simulink model "HANcoder_E407_CAN_COMM_TEST"  (R2018b)
settings: Solver=FixedStepDiscrete  StartTime=0.0  StopTime=1  FixedStep=0.01  RelTol=1e-3
PreLoadFcn:
  | librarySetup
  | eval([bdroot,'_startup']) %Calling [modelName]_startup.m
values from neighbouring files (symbols this model uses):
  HANtuneOverride = Simulink.Parameter    [HANcoder_E407_CAN_COMM_TEST_startup.m]    (also in HANcoder_E407_TTA_Controller_v3_startup.m; HANcoder_E407_TTA_Template_startup.m; HANcoder_Olimexino_startup.m)
  ID_CAN1_const = 24    [HANcoder_E407_CAN_COMM_TEST_startup.m]
  ID_CAN2_const = 24    [HANcoder_E407_CAN_COMM_TEST_startup.m]
  precision_CAN1 = Simulink.Parameter    [HANcoder_E407_CAN_COMM_TEST_startup.m]
  precision_CAN2 = Simulink.Parameter    [HANcoder_E407_CAN_COMM_TEST_startup.m]
  Rx_ID_CAN1 = Simulink.Parameter    [HANcoder_E407_CAN_COMM_TEST_startup.m]
  Rx_ID_CAN2 = Simulink.Parameter    [HANcoder_E407_CAN_COMM_TEST_startup.m]
  Tx_Buffer_1_CAN1 = Simulink.Parameter    [HANcoder_E407_CAN_COMM_TEST_startup.m]
  Tx_Buffer_1_CAN2 = Simulink.Parameter    [HANcoder_E407_CAN_COMM_TEST_startup.m]
  Tx_Buffer_2_CAN1 = Simulink.Parameter    [HANcoder_E407_CAN_COMM_TEST_startup.m]
  Tx_Buffer_2_CAN2 = Simulink.Parameter    [HANcoder_E407_CAN_COMM_TEST_startup.m]
  Tx_Buffer_3_CAN1 = Simulink.Parameter    [HANcoder_E407_CAN_COMM_TEST_startup.m]
  Tx_Buffer_3_CAN2 = Simulink.Parameter    [HANcoder_E407_CAN_COMM_TEST_startup.m]
  Tx_Buffer_4_CAN1 = Simulink.Parameter    [HANcoder_E407_CAN_COMM_TEST_startup.m]
  Tx_Buffer_4_CAN2 = Simulink.Parameter    [HANcoder_E407_CAN_COMM_TEST_startup.m]
  Tx_Buffer_5_CAN1 = Simulink.Parameter    [HANcoder_E407_CAN_COMM_TEST_startup.m]
  Tx_Buffer_5_CAN2 = Simulink.Parameter    [HANcoder_E407_CAN_COMM_TEST_startup.m]
  Tx_Buffer_6_CAN1 = Simulink.Parameter    [HANcoder_E407_CAN_COMM_TEST_startup.m]
  Tx_Buffer_6_CAN2 = Simulink.Parameter    [HANcoder_E407_CAN_COMM_TEST_startup.m]
  Tx_Buffer_7_CAN1 = Simulink.Parameter    [HANcoder_E407_CAN_COMM_TEST_startup.m]
  Tx_Buffer_7_CAN2 = Simulink.Parameter    [HANcoder_E407_CAN_COMM_TEST_startup.m]
  Tx_Buffer_8_CAN1 = Simulink.Parameter    [HANcoder_E407_CAN_COMM_TEST_startup.m]
  Tx_Buffer_8_CAN2 = Simulink.Parameter    [HANcoder_E407_CAN_COMM_TEST_startup.m]
  Tx_ID_CAN1 = Simulink.Parameter    [HANcoder_E407_CAN_COMM_TEST_startup.m]
  Tx_ID_CAN2 = Simulink.Parameter    [HANcoder_E407_CAN_COMM_TEST_startup.m]
  Tx_Max_CAN1 = Simulink.Parameter    [HANcoder_E407_CAN_COMM_TEST_startup.m]
  Tx_Max_CAN2 = Simulink.Parameter    [HANcoder_E407_CAN_COMM_TEST_startup.m]
  Tx_Min_CAN1 = Simulink.Parameter    [HANcoder_E407_CAN_COMM_TEST_startup.m]
  Tx_Min_CAN2 = Simulink.Parameter    [HANcoder_E407_CAN_COMM_TEST_startup.m]
libraries: hdlsllib x48, HANcoder_STM32_Target x13, simulink x2
(part 1 of 3)
CloseFcn:
  | rtwprivate ssgencode ModelCloseRequest mytest
settings Model: Creator=Jason van Kolfschoten  LastModifiedBy=Diego
settings SolverCC: PositivePriorityOrder=on
settings DataIOCC: LimitDataPoints=on  SaveFormat=Array  SignalLoggingSaveFormat=ModelDataLogs  SaveOutput=off  SaveTime=off
settings OptimizationCC: BlockReduction=off  DefaultParameterBehavior=Inlined  InlineInvariantSignals=on  ExpressionDepthLimit=2147483647  StateBitsets=on  DataBitsets=on  ZeroExternalMemoryAtStartup=off  ZeroInternalMemoryAtStartup=off  InitFltsAndDblsToZero=on  NoFixptDivByZeroProtection=on  EfficientFloat2IntCast=on  LifeSpan=inf
settings DebuggingCC: SaveWithDisabledLinksMsg=none  SaveWithParameterizedLinksMsg=none  CheckSSInitialOutputMsg=off  UnderspecifiedInitializationDetection=Classic  MergeDetectMultiDrivingBlocksExec=none  SignalResolutionControl=TryResolveAll  SolverPrmCheckMsg=warning  InheritedTsInSrcMsg=none  MultiTaskDSMMsg=warning  MultiTaskCondExecSysMsg=none  ParameterPrecisionLossMsg=none  FcnCallInpInsideContextMsg=warning  StateNameClashWarn=warning  SFUnexpectedBacktrackingDiag=warning  SFNoUnconditionalDefaultTransitionDiag=warning  SFExecutionAtInitializationDiag=none
settings HardwareCC: ProdBitPerPointer=32  ProdBitPerSizeT=32  ProdBitPerPtrDiffT=32  ProdLargestAtomicFloat=None  ProdIntDivRoundTo=Undefined  ProdWordSize=32  ProdHWDeviceType=Generic->32-bit Embedded Processor  TargetEndianess=LittleEndian  TargetHWDeviceType=Infineon->TriCore
settings ModelReferenceCC: PropagateSignalLabelsOutOfModel=off
settings SFSimCC: SimUseLocalCustomCode=off  MATLABDynamicMemAlloc=off
settings RTWCC: SystemTargetFile=ert.tlc  MakeCommand=make_rtw SHELL= HANcoder_PORTABLE=1 HANcoder_BOOTLOADER=1  TemplateMakefile=STM32_E407_gcc.tmf  Description=Real-Time Workshop Embedded Coder (no auto configuration)  RTWUseLocalCustomCode=off
settings CodeAppCC: ForceParamTrailComments=on  IgnoreCustomStorageClasses=off  SimulinkDataObjDesc=on  CustomSymbolStrGlobalVar=rt$N$M  CustomSymbolStrType=$N$M  CustomSymbolStrFcn=$N$M$F  CustomSymbolStrMacro=$N$M  InsertBlockDesc=on  StateflowObjectComments=on  InternalIdentifier=Classic
settings ERTTargetCC: TargetFcnLib=ansi_tfl_tmw.mat  MultiwordLength=2048  IncludeMdlTerminateFcn=off  SuppressErrorStatus=on  SupportNonFinite=off  GenerateASAP2=on  InlinedParameterPlacement=NonHierarchical  ERTCustomFileTemplate=example_file_process.tlc  ConvertIfToSwitch=off  SuppressUnreachableDefaultCases=off
settings ConfigComp: CovMetricSettings=dw  CovHtmlReporting=on  CovSaveCumulativeToWorkspaceVar=on  CovSaveSingleToWorkspaceVar=on  CovExternalEMLEnable=off  DVMaxProcessTime=600  DVDisplayUnsatisfiableObjectives=on  DVAutomaticStubbing=off  DVModelCoverageObjectives=MCDC  DVMaxTestCaseSteps=500  DVTestSuiteOptimization=CombinedObjectives  DVDetectActiveLogic=on  DVSaveHarnessModel=on

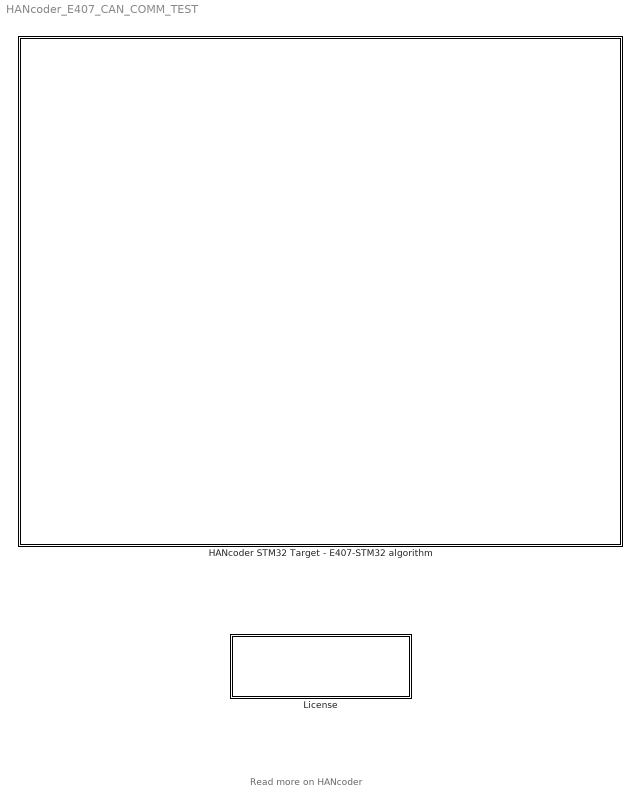
== system HANcoder_E407_CAN_COMM_TEST ==
  note: Read more on HANcoder
  HANcoder STM32 Target - E407-STM32 algorithm : Subsystem  mask(TopLevelSubsystem){}
      settings: CopyFcn=HANcoderChecks('Copy');  NameChangeFcn=HANcoderChecks('NameChangeE407');  MoveFcn=HANcoderChecks('MoveE407');
      mask Display: image(imread('STM32_E407_HAN.jpg'))
  License : Subsystem  mask(License){}
      settings: NameChangeFcn=HANcoderChecks('NameChangeLicenseBlock');  OpenFcn=winopen('License.pdf')  MoveFcn=HANcoderChecks('MoveLicenseBlock');
      mask Display: disp(['End-User License Agreement\n','please read before use']);

== system HANcoder_E407_CAN_COMM_TEST/HANcoder STM32 Target - E407-STM32 algorithm ==
  note: Board with ID 2 receives the messages
  note: Board with ID1 sends a message when the WKUP Button is pressed
  note: Basic principle:
      |
      | - Board id 1 sends a count over both CAN buses.
      |
      | - Other board receives the messages.
  note: Template model
  AND1 : Logic  IconShape=distinctive  AllPortsSameDT=off  OutDataTypeStr=boolean
  AND3 : Logic  IconShape=distinctive  AllPortsSameDT=off  OutDataTypeStr=boolean
  Algorithm : Subsystem
  Base Sample Time config : HANcoder_STM32_Target/STM32-E407/System Config/Base Sample Time config  Tag=HANcoder_TARGET_STM32_E407  Description=HANcoder Target STM32-E407 blockset version 1.0  baseSampleTime=10  extraStack=0
      settings: SourceProductName=HANcoder STM32 Target
  Build settings : HANcoder_STM32_Target/STM32-E407/System Config/Build settings  Tag=HANcoder_TARGET_STM32_E407  AutoASAP2add=on  AutoFlash=USB
      settings: SourceProductName=HANcoder STM32 Target
  CAN config : HANcoder_STM32_Target/STM32-E407/System Config/CAN config  Tag=HANcoder_TARGET_STM32_E407  txBufSize=64  evBufSize=8  canBus1=on  baudRate1=125  rxMask1=hex2dec('00000000')  rxCode1=hex2dec('00000000')  rxMode1=Receive only 11-bit message identifiers  canBus2=on  baudRate2=125  rxMask2=hex2dec('00000000')  rxCode2=hex2dec('00000000')  rxMode2=Receive only 11-bit message identifiers
      settings: SourceProductName=HANcoder STM32 Target
  Custom ID config : HANcoder_STM32_Target/STM32-E407/System Config/Custom ID config  Tag=HANcoder_TARGET_STM32_E407  softID=softwareID  softNUM=1
      settings: SourceProductName=HANcoder STM32 Target
  Data Store Memory : DataStoreMemory  DataStoreName=HANtuneOverride1  ReadBeforeWriteMsg=warning  WriteAfterWriteMsg=warning  WriteAfterReadMsg=warning  ShowAdditionalParam=off
  Digital Input : HANcoder_STM32_Target/STM32-E407/Digital Inputs/Digital Input  Tag=HANcoder_TARGET_STM32_E407  pinID=CON3 - D2 - 5V Tolerant  config=Pulldown  tsamp=-1
      settings: SourceProductName=HANcoder STM32 Target
  Digital Input1 : HANcoder_STM32_Target/STM32-E407/Digital Inputs/Digital Input  Tag=HANcoder_TARGET_STM32_E407  pinID=CON3 - D3 - 5V Tolerant  config=Pulldown  tsamp=-1
      settings: SourceProductName=HANcoder STM32 Target
  Inputs : Subsystem
  Outputs : Subsystem
  Rx CAN : Subsystem
  System information : Subsystem
  Tx CAN : Subsystem  TreatAsAtomicUnit=on
  XCP on CAN config : HANcoder_STM32_Target/STM32-E407/System Config/XCP on CAN config  Tag=HANcoder_TARGET_STM32_E407  Commented=on  canBus=CAN 1  croID=hex2dec('665')  dtoID=hex2dec('666')
      settings: SourceProductName=HANcoder STM32 Target
  XCP on USB config : HANcoder_STM32_Target/STM32-E407/System Config/XCP on USB config  Tag=HANcoder_TARGET_STM32_E407
      settings: SourceProductName=HANcoder STM32 Target
  wires:
  Inputs/1(Button) -> Algorithm/1(Button), AND1/1, AND3/1  "WKUP_button"
  Algorithm/1(LED) -> Outputs/1(LED)
  Digital Input/1 -> AND3/2  "sender_id"
  AND3/1 -> Tx CAN/Enable
  Digital Input1/1 -> AND1/2  "receiver_id"
  AND1/1 -> Rx CAN/Enable

== system HANcoder_E407_CAN_COMM_TEST/License ==

== system HANcoder_E407_CAN_COMM_TEST/HANcoder STM32 Target - E407-STM32 algorithm/Algorithm ==
  note: The button or the HANtuneOverride parameter
      | switches between the two frequencies.
  note: Here the algorithm can be placed. No hardware dependent blocks should be used here.
  note: Switch LED frequency when button is pressed
  Button : Inport
  10Hz Counter Limiter : simulink/Sources/Counter Limited  uplimit=1  tsamp=0.1
  5Hz Counter Limited : simulink/Sources/Counter Limited  uplimit=1  tsamp=0.2
  Constant : Constant  Value=HANtuneOverride  OutDataTypeStr=boolean
  Data Type Conversion : DataTypeConversion  OutDataTypeStr=boolean
  Logical Operator : Logic  Operator=OR  AllPortsSameDT=off  OutDataTypeStr=boolean
  Switch : Switch  Criteria=u2 > Threshold
  LED : Outport
  wires:
  Data Type Conversion/1 -> LED/1  "LedValue"
  5Hz Counter Limited/1 -> Switch/3
  Switch/1 -> Data Type Conversion/1
  Button/1 -> Logical Operator/2
  Logical Operator/1 -> Switch/2
  Constant/1 -> Logical Operator/1
  10Hz Counter Limiter/1 -> Switch/1

== system HANcoder_E407_CAN_COMM_TEST/HANcoder STM32 Target - E407-STM32 algorithm/Inputs ==
  note: The inputs and outputs are kept in a separate subsystem, this way the algorithm can easily be transferred to different hardware
  Digital Input : HANcoder_STM32_Target/STM32-E407/Digital Inputs/Digital Input  Tag=HANcoder_TARGET_STM32_E407  pinID=WKUP button  config=Pulldown  tsamp=-1
      settings: SourceProductName=HANcoder STM32 Target
  Button : Outport
  wires:
  Digital Input/1 -> Button/1

== system HANcoder_E407_CAN_COMM_TEST/HANcoder STM32 Target - E407-STM32 algorithm/Outputs ==
  note: The inputs and outputs are kept in a separate subsystem, this way the algorithm can easily be transferred to different hardware
  LED : Inport
  Digital Output : HANcoder_STM32_Target/STM32-E407/Digital Outputs/Digital Output  Tag=HANcoder_TARGET_STM32_E407  pinID=LED  config=Push pull  tsamp=-1
      settings: SourceProductName=HANcoder STM32 Target
  wires:
  LED/1 -> Digital Output/1

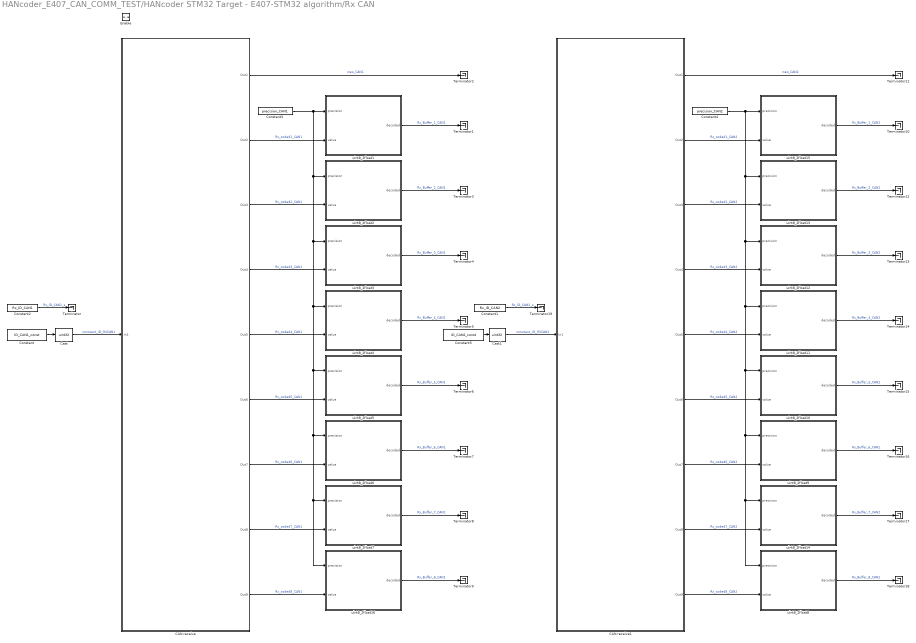
== system HANcoder_E407_CAN_COMM_TEST/HANcoder STM32 Target - E407-STM32 algorithm/Rx CAN ==
  Enable : EnablePort
  CAN receive : Subsystem  Tag=HANcoder_TARGET_STM32_E407  AncestorBlock=HANcoder_STM32_Target/STM32-E407/CAN/CAN/CAN receive  mask(CAN receive){canBus=CAN 1, outputNumber=8, dataType=uint8, byteOrder=off, tsamp=-1}
      mask prompts: canBus "CAN channel"; outputNumber "Output ports"; dataType "Output datatype"; byteOrder "Byte order: Checked = MSB first, unchecked = LSB first."; tsamp "Sample time"
      mask help:
      | Function
      | ==========
      | Receive the newest message from the specified CAN channel.
      |
      | Parameters
      | ==========
      | CAN channel:             The CAN channel to send the message on.
      | Output ports:             The amount of output ports
      | Output datatype:       The datatype of the output ports
      | Byte order:                 Select MSB or LSB first
      | Sample time:              -1 or divisible by base sample time [seconds]
      |
      | Input
      | ==========
      | Port 1:                       CAN ID(uint32) in hexadecimal ie: hex2dec('0a')
      |
      | Output
      | ==========
      | Port 1:                       Checks for new message(int8)
      | Port 2..9                     Message data
      mask init:
      | sfcn_can_receive_mcb(canBus, outputNumber, dataType, byteOrder)
      settings: MoveFcn=drawLogos
      mask Help: web('sfcn_can_receive.html');
      mask TypeOptions canBus: CAN 1 | CAN 2
      mask TypeOptions dataType: int8 | uint8 | int16 | uint16 | int32 | uint32 | boolean
      mask Display:
      | fprintf('Receive on\nCAN %x', canBus);
      | port_label('output', 1, 'new');
      | port_label('input', 1, 'ID');patch([335 341 341],[8 14 2],[1 0 0]);patch([343 343 349],[14 2 8],[0 0 0.35]);
  CAN receive1 : Subsystem  Tag=HANcoder_TARGET_STM32_E407  AncestorBlock=HANcoder_STM32_Target/STM32-E407/CAN/CAN/CAN receive  mask(CAN receive){canBus=CAN 2, outputNumber=8, dataType=uint8, byteOrder=off, tsamp=-1}
      mask prompts: canBus "CAN channel"; outputNumber "Output ports"; dataType "Output datatype"; byteOrder "Byte order: Checked = MSB first, unchecked = LSB first."; tsamp "Sample time"
      mask help:
      | Function
      | ==========
      | Receive the newest message from the specified CAN channel.
      |
      | Parameters
      | ==========
      | CAN channel:             The CAN channel to send the message on.
      | Output ports:             The amount of output ports
      | Output datatype:       The datatype of the output ports
      | Byte order:                 Select MSB or LSB first
      | Sample time:              -1 or divisible by base sample time [seconds]
      |
      | Input
      | ==========
      | Port 1:                       CAN ID(uint32) in hexadecimal ie: hex2dec('0a')
      |
      | Output
      | ==========
      | Port 1:                       Checks for new message(int8)
      | Port 2..9                     Message data
      mask init:
      | sfcn_can_receive_mcb(canBus, outputNumber, dataType, byteOrder)
      settings: MoveFcn=drawLogos
      mask Help: web('sfcn_can_receive.html');
      mask TypeOptions canBus: CAN 1 | CAN 2
      mask TypeOptions dataType: int8 | uint8 | int16 | uint16 | int32 | uint32 | boolean
      mask Display:
      | fprintf('Receive on\nCAN %x', canBus);
      | port_label('output', 1, 'new');
      | port_label('input', 1, 'ID');patch([335 341 341],[8 14 2],[1 0 0]);patch([343 343 349],[14 2 8],[0 0 0.35]);
  Cast : DataTypeConversion  OutDataTypeStr=uint32
  Cast1 : DataTypeConversion  OutDataTypeStr=uint32
  Constant : Constant  Value=ID_CAN1_const
  Constant1 : Constant  Value=Rx_ID_CAN2  OutDataTypeStr=uint32
  Constant2 : Constant  Value=Rx_ID_CAN1  OutDataTypeStr=uint32
  Constant3 : Constant  Value=precision_CAN1
  Constant4 : Constant  Value=precision_CAN2
  Constant5 : Constant  Value=ID_CAN2_const
  Terminator{,1..19} (20 alike) : Terminator
  uint8_2float1 : Subsystem
  uint8_2float10 : Subsystem
  uint8_2float11 : Subsystem
  uint8_2float12 : Subsystem
  uint8_2float13 : Subsystem
  uint8_2float14 : Subsystem
  uint8_2float15 : Subsystem
  uint8_2float16 : Subsystem
  uint8_2float2 : Subsystem
  uint8_2float3 : Subsystem
  uint8_2float4 : Subsystem
  uint8_2float5 : Subsystem
  uint8_2float6 : Subsystem
  uint8_2float7 : Subsystem
  uint8_2float8 : Subsystem
  uint8_2float9 : Subsystem
  wires:
  Constant/1 -> Cast/1
  CAN receive/1(Out1) -> Terminator2/1  "new_CAN1"
  Constant3/1 -> uint8_2float1/1(precision), uint8_2float2/1(precision), uint8_2float16/1(precision), uint8_2float7/1(precision), uint8_2float6/1(precision), uint8_2float5/1(precision), uint8_2float4/1(precision), uint8_2float3/1(precision)
  CAN receive/2(Out2) -> uint8_2float1/2(value)  "Rx_coded1_CAN1"
  CAN receive/3(Out3) -> uint8_2float2/2(value)  "Rx_coded2_CAN1"
  uint8_2float1/1(decoded) -> Terminator1/1  "Rx_Buffer_1_CAN1"
  uint8_2float2/1(decoded) -> Terminator3/1  "Rx_Buffer_2_CAN1"
  uint8_2float3/1(decoded) -> Terminator4/1  "Rx_Buffer_3_CAN1"
  uint8_2float4/1(decoded) -> Terminator5/1  "Rx_Buffer_4_CAN1"
  uint8_2float5/1(decoded) -> Terminator6/1  "Rx_Buffer_5_CAN1"
  uint8_2float6/1(decoded) -> Terminator7/1  "Rx_Buffer_6_CAN1"
  uint8_2float7/1(decoded) -> Terminator8/1  "Rx_Buffer_7_CAN1"
  uint8_2float16/1(decoded) -> Terminator9/1  "Rx_Buffer_8_CAN1"
  CAN receive/9(Out9) -> uint8_2float16/2(value)  "Rx_coded8_CAN1"
  CAN receive/8(Out8) -> uint8_2float7/2(value)  "Rx_coded7_CAN1"
  CAN receive/7(Out7) -> uint8_2float6/2(value)  "Rx_coded6_CAN1"
  CAN receive/6(Out6) -> uint8_2float5/2(value)  "Rx_coded5_CAN1"
  CAN receive/5(Out5) -> uint8_2float4/2(value)  "Rx_coded4_CAN1"
  CAN receive/4(Out4) -> uint8_2float3/2(value)  "Rx_coded3_CAN1"
  CAN receive1/4(Out4) -> uint8_2float12/2(value)  "Rx_coded3_CAN2"
  CAN receive1/5(Out5) -> uint8_2float11/2(value)  "Rx_coded4_CAN2"
  CAN receive1/6(Out6) -> uint8_2float10/2(value)  "Rx_coded5_CAN2"
  CAN receive1/7(Out7) -> uint8_2float9/2(value)  "Rx_coded6_CAN2"
  CAN receive1/8(Out8) -> uint8_2float14/2(value)  "Rx_coded7_CAN2"
  CAN receive1/9(Out9) -> uint8_2float8/2(value)  "Rx_coded8_CAN2"
  uint8_2float8/1(decoded) -> Terminator18/1  "Rx_Buffer_8_CAN2"
  uint8_2float14/1(decoded) -> Terminator17/1  "Rx_Buffer_7_CAN2"
  uint8_2float9/1(decoded) -> Terminator16/1  "Rx_Buffer_6_CAN2"
  uint8_2float10/1(decoded) -> Terminator15/1  "Rx_Buffer_5_CAN2"
  uint8_2float11/1(decoded) -> Terminator14/1  "Rx_Buffer_4_CAN2"
  uint8_2float12/1(decoded) -> Terminator13/1  "Rx_Buffer_3_CAN2"
  uint8_2float13/1(decoded) -> Terminator12/1  "Rx_Buffer_2_CAN2"
  uint8_2float15/1(decoded) -> Terminator10/1  "Rx_Buffer_1_CAN2"
  CAN receive1/3(Out3) -> uint8_2float13/2(value)  "Rx_coded2_CAN2"
  CAN receive1/2(Out2) -> uint8_2float15/2(value)  "Rx_coded1_CAN2"
  Constant4/1 -> uint8_2float15/1(precision), uint8_2float13/1(precision), uint8_2float12/1(precision), uint8_2float11/1(precision), uint8_2float10/1(precision), uint8_2float9/1(precision), uint8_2float8/1(precision), uint8_2float14/1(precision)
  CAN receive1/1(Out1) -> Terminator11/1  "new_CAN2"
  Constant5/1 -> Cast1/1
  Constant2/1 -> Terminator/1  "Rx_ID_CAN1_s"
  Constant1/1 -> Terminator19/1  "Rx_ID_CAN2_s"
  Cast/1 -> CAN receive/1(In1)  "constant_ID_RXCAN1"
  Cast1/1 -> CAN receive1/1(In1)  "constant_ID_RXCAN2"

== system HANcoder_E407_CAN_COMM_TEST/HANcoder STM32 Target - E407-STM32 algorithm/System information ==
  note: These blocks check the free memory: stack and heap and the CPU load,
      | this way you can see whether your software demands too much of the microcontroller
  Get CPU load : HANcoder_STM32_Target/STM32-E407/System Management/Get CPU load  Tag=HANcoder_TARGET_STM32_E407  mode=Current CPU load  tsamp=-1
      settings: SourceProductName=HANcoder STM32 Target
  Get free Heap : HANcoder_STM32_Target/STM32-E407/System Management/Get free Heap  Tag=HANcoder_TARGET_STM32_E407  tsamp=-1
      settings: SourceProductName=HANcoder STM32 Target
  Get free Stack : HANcoder_STM32_Target/STM32-E407/System Management/Get free Stack  Tag=HANcoder_TARGET_STM32_E407  taskIdx=Application Control Task  tsamp=-1
      settings: SourceProductName=HANcoder STM32 Target
  Terminator : Terminator
  Terminator1 : Terminator
  Terminator2 : Terminator
  wires:
  Get CPU load/1 -> Terminator1/1  "SI_CPUload"
  Get free Stack/1 -> Terminator/1  "SI_FreeStack"
  Get free Heap/1 -> Terminator2/1  "SI_FreeHeap"

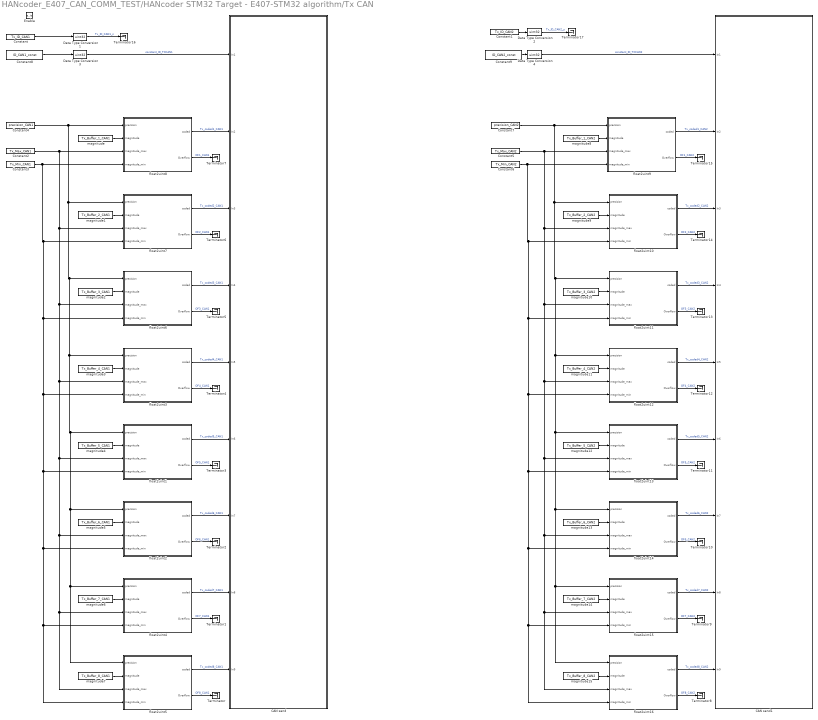
== system HANcoder_E407_CAN_COMM_TEST/HANcoder STM32 Target - E407-STM32 algorithm/Tx CAN ==
  Enable : EnablePort
  CAN send : Subsystem  Tag=HANcoder_TARGET_STM32_E407  AncestorBlock=HANcoder_STM32_Target/STM32-E407/CAN/CAN/CAN send  mask(CAN send){canBus=CAN 1, frameType=Standard (11 bit), inputNumber=8, dataType=uint8, byteOrder=off, tsamp=-1}
      mask prompts: canBus "CAN channel"; frameType "Identifier type"; inputNumber "Input ports"; dataType "Input datatype"; byteOrder "Byte order: Checked = MSB first, unchecked = LSB first."; tsamp "Sample time"
      mask help:
      | Function
      | ==========
      | Send a message on the CAN channel.
      |
      | Parameters
      | ==========
      | CAN channel:           The CAN channel to send the message on.
      | Identifier type:         normal or extended ID's
      | Input ports:              The amount of input ports
      | Input datatype:        The datatype of the input ports
      | Byte order:               Select MSB or LSB first
      | Sample time:            -1 or divisible by base sample time [seconds]
      |
      | Input
      | ==========
      | Port 1:                   CAN ID(uint32) in hexadecimal ie: hex2dec('0a')
      | Port 2..9                CAN message data
      mask init:
      | sfcn_can_send_mcb(canBus, frameType, inputNumber, dataType, byteOrder)
      settings: MoveFcn=drawLogos
      mask Help: web('sfcn_can_send.html');
      mask TypeOptions canBus: CAN 1 | CAN 2
      mask TypeOptions frameType: Standard (11 bit) | Extended (29 bit)
      mask TypeOptions dataType: int8 | uint8 | int16 | uint16 | int32 | uint32 | boolean
      mask Display:
      | fprintf('Send on\nCAN %x', canBus);
      | port_label('input', 1, 'ID');patch([280 286 286],[8 14 2],[1 0 0]);patch([288 288 294],[14 2 8],[0 0 0.35]);
  CAN send1 : Subsystem  Tag=HANcoder_TARGET_STM32_E407  AncestorBlock=HANcoder_STM32_Target/STM32-E407/CAN/CAN/CAN send  mask(CAN send){canBus=CAN 2, frameType=Standard (11 bit), inputNumber=8, dataType=uint8, byteOrder=off, tsamp=-1}
      mask prompts: canBus "CAN channel"; frameType "Identifier type"; inputNumber "Input ports"; dataType "Input datatype"; byteOrder "Byte order: Checked = MSB first, unchecked = LSB first."; tsamp "Sample time"
      mask help:
      | Function
      | ==========
      | Send a message on the CAN channel.
      |
      | Parameters
      | ==========
      | CAN channel:           The CAN channel to send the message on.
      | Identifier type:         normal or extended ID's
      | Input ports:              The amount of input ports
      | Input datatype:        The datatype of the input ports
      | Byte order:               Select MSB or LSB first
      | Sample time:            -1 or divisible by base sample time [seconds]
      |
      | Input
      | ==========
      | Port 1:                   CAN ID(uint32) in hexadecimal ie: hex2dec('0a')
      | Port 2..9                CAN message data
      mask init:
      | sfcn_can_send_mcb(canBus, frameType, inputNumber, dataType, byteOrder)
      settings: MoveFcn=drawLogos
      mask Help: web('sfcn_can_send.html');
      mask TypeOptions canBus: CAN 1 | CAN 2
      mask TypeOptions frameType: Standard (11 bit) | Extended (29 bit)
      mask TypeOptions dataType: int8 | uint8 | int16 | uint16 | int32 | uint32 | boolean
      mask Display:
      | fprintf('Send on\nCAN %x', canBus);
      | port_label('input', 1, 'ID');patch([280 286 286],[8 14 2],[1 0 0]);patch([288 288 294],[14 2 8],[0 0 0.35]);
  Constant : Constant  Value=Tx_ID_CAN1
  Constant1 : Constant  Value=Tx_ID_CAN2
  Constant2 : Constant  Value=Tx_Max_CAN1
  Constant3 : Constant  Value=Tx_Min_CAN1
  Constant4 : Constant  Value=precision_CAN1
  Constant5 : Constant  Value=Tx_Max_CAN2
  Constant6 : Constant  Value=Tx_Min_CAN2
  Constant7 : Constant  Value=precision_CAN2
  Constant8 : Constant  Value=ID_CAN1_const
  Constant9 : Constant  Value=ID_CAN2_const
  Data Type Conversion{1..4} (4 alike) : DataTypeConversion  OutDataTypeStr=uint32
  Terminator{,1..17} (18 alike) : Terminator
  float2uint1 : Subsystem
  float2uint10 : Subsystem
  float2uint11 : Subsystem
  float2uint12 : Subsystem
  float2uint13 : Subsystem
  float2uint14 : Subsystem
  float2uint15 : Subsystem
  float2uint16 : Subsystem
  float2uint2 : Subsystem
  float2uint3 : Subsystem
  float2uint4 : Subsystem
  float2uint5 : Subsystem
  float2uint6 : Subsystem
  float2uint7 : Subsystem
  float2uint8 : Subsystem
  float2uint9 : Subsystem
  magnitude : Constant  Value=Tx_Buffer_1_CAN1
  magnitude1 : Constant  Value=Tx_Buffer_2_CAN1
  magnitude10 : Constant  Value=Tx_Buffer_3_CAN2
  magnitude11 : Constant  Value=Tx_Buffer_4_CAN2
  magnitude12 : Constant  Value=Tx_Buffer_5_CAN2
  magnitude13 : Constant  Value=Tx_Buffer_6_CAN2
  magnitude14 : Constant  Value=Tx_Buffer_7_CAN2
  magnitude15 : Constant  Value=Tx_Buffer_8_CAN2
  magnitude2 : Constant  Value=Tx_Buffer_3_CAN1
  magnitude3 : Constant  Value=Tx_Buffer_4_CAN1
  magnitude4 : Constant  Value=Tx_Buffer_5_CAN1
  magnitude5 : Constant  Value=Tx_Buffer_6_CAN1
  magnitude6 : Constant  Value=Tx_Buffer_7_CAN1
  magnitude7 : Constant  Value=Tx_Buffer_8_CAN1
  magnitude8 : Constant  Value=Tx_Buffer_1_CAN2
  magnitude9 : Constant  Value=Tx_Buffer_2_CAN2
  wires:
  Constant8/1 -> Data Type Conversion3/1
  Constant/1 -> Data Type Conversion1/1
  Constant3/1 -> float2uint8/4(magnitude_min), float2uint7/4(magnitude_min), float2uint6/4(magnitude_min), float2uint1/4(magnitude_min), float2uint2/4(magnitude_min), float2uint5/4(magnitude_min), float2uint4/4(magnitude_min), float2uint3/4(magnitude_min)
  Constant2/1 -> float2uint8/3(magnitude_max), float2uint7/3(magnitude_max), float2uint6/3(magnitude_max), float2uint1/3(magnitude_max), float2uint2/3(magnitude_max), float2uint5/3(magnitude_max), float2uint4/3(magnitude_max), float2uint3/3(magnitude_max)
  Constant4/1 -> float2uint8/1(precision), float2uint7/1(precision), float2uint6/1(precision), float2uint1/1(precision), float2uint2/1(precision), float2uint5/1(precision), float2uint4/1(precision), float2uint3/1(precision)
  magnitude/1 -> float2uint8/2(magnitude)
  magnitude1/1 -> float2uint7/2(magnitude)
  magnitude2/1 -> float2uint6/2(magnitude)
  magnitude3/1 -> float2uint3/2(magnitude)
  magnitude4/1 -> float2uint1/2(magnitude)
  magnitude5/1 -> float2uint2/2(magnitude)
  magnitude6/1 -> float2uint4/2(magnitude)
  magnitude7/1 -> float2uint5/2(magnitude)
  float2uint8/1(coded) -> CAN send/2(In2)  "Tx_coded1_CAN1"
  float2uint7/1(coded) -> CAN send/3(In3)  "Tx_coded2_CAN1"
  float2uint6/1(coded) -> CAN send/4(In4)  "Tx_coded3_CAN1"
  float2uint3/1(coded) -> CAN send/5(In5)  "Tx_coded4_CAN1"
  float2uint1/1(coded) -> CAN send/6(In6)  "Tx_coded5_CAN1"
  float2uint2/1(coded) -> CAN send/7(In7)  "Tx_coded6_CAN1"
  float2uint4/1(coded) -> CAN send/8(In8)  "Tx_coded7_CAN1"
  float2uint5/1(coded) -> CAN send/9(In9)  "Tx_coded8_CAN1"
  float2uint5/2(Overflow) -> Terminator/1  "OF8_CAN1"
  float2uint4/2(Overflow) -> Terminator1/1  "OF7_CAN1"
  float2uint2/2(Overflow) -> Terminator2/1  "OF6_CAN1"
  float2uint1/2(Overflow) -> Terminator3/1  "OF5_CAN1"
  float2uint3/2(Overflow) -> Terminator4/1  "OF4_CAN1"
  float2uint6/2(Overflow) -> Terminator5/1  "OF3_CAN1"
  float2uint7/2(Overflow) -> Terminator6/1  "OF2_CAN1"
  float2uint8/2(Overflow) -> Terminator7/1  "OF1_CAN1"
  float2uint9/2(Overflow) -> Terminator15/1  "OF1_CAN2"
  float2uint10/2(Overflow) -> Terminator14/1  "OF2_CAN2"
  float2uint11/2(Overflow) -> Terminator13/1  "OF3_CAN2"
  float2uint12/2(Overflow) -> Terminator12/1  "OF4_CAN2"
  float2uint13/2(Overflow) -> Terminator11/1  "OF5_CAN2"
  float2uint14/2(Overflow) -> Terminator10/1  "OF6_CAN2"
  float2uint15/2(Overflow) -> Terminator9/1  "OF7_CAN2"
  float2uint16/2(Overflow) -> Terminator8/1  "OF8_CAN2"
  float2uint16/1(coded) -> CAN send1/9(In9)  "Tx_coded8_CAN2"
  float2uint15/1(coded) -> CAN send1/8(In8)  "Tx_coded7_CAN2"
  float2uint14/1(coded) -> CAN send1/7(In7)  "Tx_coded6_CAN2"
  float2uint13/1(coded) -> CAN send1/6(In6)  "Tx_coded5_CAN2"
  float2uint12/1(coded) -> CAN send1/5(In5)  "Tx_coded4_CAN2"
  float2uint11/1(coded) -> CAN send1/4(In4)  "Tx_coded3_CAN2"
  float2uint10/1(coded) -> CAN send1/3(In3)  "Tx_coded2_CAN2"
  float2uint9/1(coded) -> CAN send1/2(In2)  "Tx_coded1_CAN2"
  magnitude15/1 -> float2uint16/2(magnitude)
  magnitude14/1 -> float2uint15/2(magnitude)
  magnitude13/1 -> float2uint14/2(magnitude)
  magnitude12/1 -> float2uint13/2(magnitude)
  magnitude11/1 -> float2uint12/2(magnitude)
  magnitude10/1 -> float2uint11/2(magnitude)
  magnitude9/1 -> float2uint10/2(magnitude)
  magnitude8/1 -> float2uint9/2(magnitude)
  Constant7/1 -> float2uint9/1(precision), float2uint10/1(precision), float2uint11/1(precision), float2uint12/1(precision), float2uint13/1(precision), float2uint14/1(precision), float2uint16/1(precision), float2uint15/1(precision)
  Constant5/1 -> float2uint9/3(magnitude_max), float2uint10/3(magnitude_max), float2uint11/3(magnitude_max), float2uint12/3(magnitude_max), float2uint13/3(magnitude_max), float2uint14/3(magnitude_max), float2uint16/3(magnitude_max), float2uint15/3(magnitude_max)
  Constant6/1 -> float2uint9/4(magnitude_min), float2uint10/4(magnitude_min), float2uint11/4(magnitude_min), float2uint12/4(magnitude_min), float2uint13/4(magnitude_min), float2uint14/4(magnitude_min), float2uint16/4(magnitude_min), float2uint15/4(magnitude_min)
  Constant1/1 -> Data Type Conversion2/1
  Data Type Conversion4/1 -> CAN send1/1(In1)  "constant_ID_TXCAN2"
  Data Type Conversion1/1 -> Terminator16/1  "Tx_ID_CAN1_s"
  Data Type Conversion3/1 -> CAN send/1(In1)  "constant_ID_TXCAN1"
  Constant9/1 -> Data Type Conversion4/1
  Data Type Conversion2/1 -> Terminator17/1  "Tx_ID_CAN2_s"

== system HANcoder_E407_CAN_COMM_TEST/HANcoder STM32 Target - E407-STM32 algorithm/Rx CAN/CAN receive ==
  In1 : Inport
  Enabled Subsystem : Subsystem  TreatAsAtomicUnit=on
  S-Function : M-S-Function  FunctionName=sfcn_can_receive  Parameters=tsamp, canBus, outputNumber, dataType, byteOrder
  Out1 : Outport
  Out2 : Outport  Port=2
  Out3 : Outport  Port=3
  Out4 : Outport  Port=4
  Out5 : Outport  Port=5
  Out6 : Outport  Port=6
  Out7 : Outport  Port=7
  Out8 : Outport  Port=8
  Out9 : Outport  Port=9
  wires:
  S-Function/9 -> Enabled Subsystem/8(In8)
  S-Function/4 -> Enabled Subsystem/3(In3)
  S-Function/5 -> Enabled Subsystem/4(In4)
  S-Function/8 -> Enabled Subsystem/7(In7)
  S-Function/7 -> Enabled Subsystem/6(In6)
  S-Function/6 -> Enabled Subsystem/5(In5)
  Enabled Subsystem/8(Out8) -> Out9/1
  Enabled Subsystem/7(Out7) -> Out8/1
  Enabled Subsystem/6(Out6) -> Out7/1
  Enabled Subsystem/5(Out5) -> Out6/1
  Enabled Subsystem/4(Out4) -> Out5/1
  Enabled Subsystem/3(Out3) -> Out4/1
  Enabled Subsystem/2(Out2) -> Out3/1
  Enabled Subsystem/1(Out1) -> Out2/1
  S-Function/3 -> Enabled Subsystem/2(In2)
  S-Function/2 -> Enabled Subsystem/1(In1)
  S-Function/1 -> Out1/1, Enabled Subsystem/Enable
  In1/1 -> S-Function/1

== system HANcoder_E407_CAN_COMM_TEST/HANcoder STM32 Target - E407-STM32 algorithm/Rx CAN/CAN receive1 ==
  In1 : Inport
  Enabled Subsystem : Subsystem  TreatAsAtomicUnit=on
  S-Function : M-S-Function  FunctionName=sfcn_can_receive  Parameters=tsamp, canBus, outputNumber, dataType, byteOrder
  Out1 : Outport
  Out2 : Outport  Port=2
  Out3 : Outport  Port=3
  Out4 : Outport  Port=4
  Out5 : Outport  Port=5
  Out6 : Outport  Port=6
  Out7 : Outport  Port=7
  Out8 : Outport  Port=8
  Out9 : Outport  Port=9
  wires:
  In1/1 -> S-Function/1
  S-Function/1 -> Enabled Subsystem/Enable, Out1/1
  S-Function/2 -> Enabled Subsystem/1(In1)
  S-Function/3 -> Enabled Subsystem/2(In2)
  Enabled Subsystem/1(Out1) -> Out2/1
  Enabled Subsystem/2(Out2) -> Out3/1
  Enabled Subsystem/3(Out3) -> Out4/1
  Enabled Subsystem/4(Out4) -> Out5/1
  Enabled Subsystem/5(Out5) -> Out6/1
  Enabled Subsystem/6(Out6) -> Out7/1
  Enabled Subsystem/7(Out7) -> Out8/1
  Enabled Subsystem/8(Out8) -> Out9/1
  S-Function/6 -> Enabled Subsystem/5(In5)
  S-Function/7 -> Enabled Subsystem/6(In6)
  S-Function/8 -> Enabled Subsystem/7(In7)
  S-Function/5 -> Enabled Subsystem/4(In4)
  S-Function/4 -> Enabled Subsystem/3(In3)
  S-Function/9 -> Enabled Subsystem/8(In8)

== system HANcoder_E407_CAN_COMM_TEST/HANcoder STM32 Target - E407-STM32 algorithm/Rx CAN/uint8_2float1 ==
  precision : Inport
  value : Inport  Port=2
  Bit Shift : hdlsllib/Logic and Bit Operations/Bit Shift  mode=Shift Right Logical  N=7
      settings: SourceProductName=HDL Coder  SourceProductBaseCode=HD
  Bit Shift1 : hdlsllib/Logic and Bit Operations/Bit Shift  mode=Shift Left Logical  N=7
      settings: SourceProductName=HDL Coder  SourceProductBaseCode=HD
  Cast1 : DataTypeConversion  OutDataTypeStr=double
  Constant1 : Constant  Value=2
  Constant2 : Constant  Value=2
  Display{1..5} (5 alike) : Display
  Divide : Product  Inputs=*/
  Fix1 : Rounding  Operator=fix
  Gain : Gain  Gain=-1
  Gain1 : Gain  Gain=-1
  Minus : Sum  Inputs=-+
  Minus1 : Sum  Inputs=+-
  Minus2 : Sum
  Multiply : Product
  Multiply1 : Product
  Power : Math  Priority=5  Operator=pow  SaturateOnIntegerOverflow=on
  Power1 : Math  Priority=5  Operator=pow  SaturateOnIntegerOverflow=on
  Switch : Switch  Criteria=u2 > Threshold
  decoded : Outport
  wires:
  Bit Shift/1 -> Bit Shift1/1, Switch/2, Display1/1
  value/1 -> Cast1/1, Bit Shift/1
  Minus/1 -> Divide/1, Display2/1, Minus1/1
  Fix1/1 -> Minus2/2, Display4/1, Multiply1/1
  Multiply1/1 -> Minus1/2
  Minus1/1 -> Display5/1, Multiply/1
  Constant1/1 -> Power/1
  Gain/1 -> Power/2
  Power/1 -> Multiply/2
  [precision] -> Gain/1
  Multiply/1 -> Minus2/1
  Minus2/1 -> Gain1/1, Switch/3
  Gain1/1 -> Switch/1
  Switch/1 -> Display3/1, decoded/1
  Divide/1 -> Fix1/1
  Cast1/1 -> Minus/2
  precision/1 -> Power1/2, [precision]
  Constant2/1 -> Power1/1
  Power1/1 -> [prec_pow]
  [prec_pow] -> Divide/2
  [prec_pow] -> Multiply1/2
  Bit Shift1/1 -> Minus/1

== system HANcoder_E407_CAN_COMM_TEST/HANcoder STM32 Target - E407-STM32 algorithm/Rx CAN/uint8_2float10 ==
  precision : Inport
  value : Inport  Port=2
  Bit Shift : hdlsllib/Logic and Bit Operations/Bit Shift  mode=Shift Right Logical  N=7
      settings: SourceProductName=HDL Coder  SourceProductBaseCode=HD
  Bit Shift1 : hdlsllib/Logic and Bit Operations/Bit Shift  mode=Shift Left Logical  N=7
      settings: SourceProductName=HDL Coder  SourceProductBaseCode=HD
  Cast1 : DataTypeConversion  OutDataTypeStr=double
  Constant1 : Constant  Value=2
  Constant2 : Constant  Value=2
  Display{1..5} (5 alike) : Display
  Divide : Product  Inputs=*/
  Fix1 : Rounding  Operator=fix
  Gain : Gain  Gain=-1
  Gain1 : Gain  Gain=-1
  Minus : Sum  Inputs=-+
  Minus1 : Sum  Inputs=+-
  Minus2 : Sum
  Multiply : Product
  Multiply1 : Product
  Power : Math  Priority=5  Operator=pow  SaturateOnIntegerOverflow=on
  Power1 : Math  Priority=5  Operator=pow  SaturateOnIntegerOverflow=on
  Switch : Switch  Criteria=u2 > Threshold
  decoded : Outport
  wires:
  Bit Shift1/1 -> Minus/1
  [prec_pow] -> Multiply1/2
  [prec_pow] -> Divide/2
  Power1/1 -> [prec_pow]
  Constant2/1 -> Power1/1
  precision/1 -> [precision], Power1/2
  Cast1/1 -> Minus/2
  Divide/1 -> Fix1/1
  Switch/1 -> decoded/1, Display3/1
  Gain1/1 -> Switch/1
  Minus2/1 -> Switch/3, Gain1/1
  Multiply/1 -> Minus2/1
  [precision] -> Gain/1
  Power/1 -> Multiply/2
  Gain/1 -> Power/2
  Constant1/1 -> Power/1
  Minus1/1 -> Multiply/1, Display5/1
  Multiply1/1 -> Minus1/2
  Fix1/1 -> Multiply1/1, Display4/1, Minus2/2
  Minus/1 -> Minus1/1, Display2/1, Divide/1
  value/1 -> Bit Shift/1, Cast1/1
  Bit Shift/1 -> Display1/1, Switch/2, Bit Shift1/1

== system HANcoder_E407_CAN_COMM_TEST/HANcoder STM32 Target - E407-STM32 algorithm/Rx CAN/uint8_2float11 ==
  precision : Inport
  value : Inport  Port=2
  Bit Shift : hdlsllib/Logic and Bit Operations/Bit Shift  mode=Shift Right Logical  N=7
      settings: SourceProductName=HDL Coder  SourceProductBaseCode=HD
  Bit Shift1 : hdlsllib/Logic and Bit Operations/Bit Shift  mode=Shift Left Logical  N=7
      settings: SourceProductName=HDL Coder  SourceProductBaseCode=HD
  Cast1 : DataTypeConversion  OutDataTypeStr=double
  Constant1 : Constant  Value=2
  Constant2 : Constant  Value=2
  Display{1..5} (5 alike) : Display
  Divide : Product  Inputs=*/
  Fix1 : Rounding  Operator=fix
  Gain : Gain  Gain=-1
  Gain1 : Gain  Gain=-1
  Minus : Sum  Inputs=-+
  Minus1 : Sum  Inputs=+-
  Minus2 : Sum
  Multiply : Product
  Multiply1 : Product
  Power : Math  Priority=5  Operator=pow  SaturateOnIntegerOverflow=on
  Power1 : Math  Priority=5  Operator=pow  SaturateOnIntegerOverflow=on
  Switch : Switch  Criteria=u2 > Threshold
  decoded : Outport
  wires:
  Bit Shift/1 -> Bit Shift1/1, Switch/2, Display1/1
  value/1 -> Cast1/1, Bit Shift/1
  Minus/1 -> Divide/1, Display2/1, Minus1/1
  Fix1/1 -> Minus2/2, Display4/1, Multiply1/1
  Multiply1/1 -> Minus1/2
  Minus1/1 -> Display5/1, Multiply/1
  Constant1/1 -> Power/1
  Gain/1 -> Power/2
  Power/1 -> Multiply/2
  [precision] -> Gain/1
  Multiply/1 -> Minus2/1
  Minus2/1 -> Gain1/1, Switch/3
  Gain1/1 -> Switch/1
  Switch/1 -> Display3/1, decoded/1
  Divide/1 -> Fix1/1
  Cast1/1 -> Minus/2
  precision/1 -> Power1/2, [precision]
  Constant2/1 -> Power1/1
  Power1/1 -> [prec_pow]
  [prec_pow] -> Divide/2
  [prec_pow] -> Multiply1/2
  Bit Shift1/1 -> Minus/1

== system HANcoder_E407_CAN_COMM_TEST/HANcoder STM32 Target - E407-STM32 algorithm/Rx CAN/uint8_2float12 ==
  precision : Inport
  value : Inport  Port=2
  Bit Shift : hdlsllib/Logic and Bit Operations/Bit Shift  mode=Shift Right Logical  N=7
      settings: SourceProductName=HDL Coder  SourceProductBaseCode=HD
  Bit Shift1 : hdlsllib/Logic and Bit Operations/Bit Shift  mode=Shift Left Logical  N=7
      settings: SourceProductName=HDL Coder  SourceProductBaseCode=HD
  Cast1 : DataTypeConversion  OutDataTypeStr=double
  Constant1 : Constant  Value=2
  Constant2 : Constant  Value=2
  Display{1..5} (5 alike) : Display
  Divide : Product  Inputs=*/
  Fix1 : Rounding  Operator=fix
  Gain : Gain  Gain=-1
  Gain1 : Gain  Gain=-1
  Minus : Sum  Inputs=-+
  Minus1 : Sum  Inputs=+-
  Minus2 : Sum
  Multiply : Product
  Multiply1 : Product
  Power : Math  Priority=5  Operator=pow  SaturateOnIntegerOverflow=on
  Power1 : Math  Priority=5  Operator=pow  SaturateOnIntegerOverflow=on
  Switch : Switch  Criteria=u2 > Threshold
  decoded : Outport
  wires:
  Bit Shift1/1 -> Minus/1
  [prec_pow] -> Multiply1/2
  [prec_pow] -> Divide/2
  Power1/1 -> [prec_pow]
  Constant2/1 -> Power1/1
  precision/1 -> [precision], Power1/2
  Cast1/1 -> Minus/2
  Divide/1 -> Fix1/1
  Switch/1 -> decoded/1, Display3/1
  Gain1/1 -> Switch/1
  Minus2/1 -> Switch/3, Gain1/1
  Multiply/1 -> Minus2/1
  [precision] -> Gain/1
  Power/1 -> Multiply/2
  Gain/1 -> Power/2
  Constant1/1 -> Power/1
  Minus1/1 -> Multiply/1, Display5/1
  Multiply1/1 -> Minus1/2
  Fix1/1 -> Multiply1/1, Display4/1, Minus2/2
  Minus/1 -> Minus1/1, Display2/1, Divide/1
  value/1 -> Bit Shift/1, Cast1/1
  Bit Shift/1 -> Display1/1, Switch/2, Bit Shift1/1

== system HANcoder_E407_CAN_COMM_TEST/HANcoder STM32 Target - E407-STM32 algorithm/Rx CAN/uint8_2float13 ==
  precision : Inport
  value : Inport  Port=2
  Bit Shift : hdlsllib/Logic and Bit Operations/Bit Shift  mode=Shift Right Logical  N=7
      settings: SourceProductName=HDL Coder  SourceProductBaseCode=HD
  Bit Shift1 : hdlsllib/Logic and Bit Operations/Bit Shift  mode=Shift Left Logical  N=7
      settings: SourceProductName=HDL Coder  SourceProductBaseCode=HD
  Cast1 : DataTypeConversion  OutDataTypeStr=double
  Constant1 : Constant  Value=2
  Constant2 : Constant  Value=2
  Display{1..5} (5 alike) : Display
  Divide : Product  Inputs=*/
  Fix1 : Rounding  Operator=fix
  Gain : Gain  Gain=-1
  Gain1 : Gain  Gain=-1
  Minus : Sum  Inputs=-+
  Minus1 : Sum  Inputs=+-
  Minus2 : Sum
  Multiply : Product
  Multiply1 : Product
  Power : Math  Priority=5  Operator=pow  SaturateOnIntegerOverflow=on
  Power1 : Math  Priority=5  Operator=pow  SaturateOnIntegerOverflow=on
  Switch : Switch  Criteria=u2 > Threshold
  decoded : Outport
  wires:
  Bit Shift/1 -> Bit Shift1/1, Switch/2, Display1/1
  value/1 -> Cast1/1, Bit Shift/1
  Minus/1 -> Divide/1, Display2/1, Minus1/1
  Fix1/1 -> Minus2/2, Display4/1, Multiply1/1
  Multiply1/1 -> Minus1/2
  Minus1/1 -> Display5/1, Multiply/1
  Constant1/1 -> Power/1
  Gain/1 -> Power/2
  Power/1 -> Multiply/2
  [precision] -> Gain/1
  Multiply/1 -> Minus2/1
  Minus2/1 -> Gain1/1, Switch/3
  Gain1/1 -> Switch/1
  Switch/1 -> Display3/1, decoded/1
  Divide/1 -> Fix1/1
  Cast1/1 -> Minus/2
  precision/1 -> Power1/2, [precision]
  Constant2/1 -> Power1/1
  Power1/1 -> [prec_pow]
  [prec_pow] -> Divide/2
  [prec_pow] -> Multiply1/2
  Bit Shift1/1 -> Minus/1

== system HANcoder_E407_CAN_COMM_TEST/HANcoder STM32 Target - E407-STM32 algorithm/Rx CAN/uint8_2float14 ==
  precision : Inport
  value : Inport  Port=2
  Bit Shift : hdlsllib/Logic and Bit Operations/Bit Shift  mode=Shift Right Logical  N=7
      settings: SourceProductName=HDL Coder  SourceProductBaseCode=HD
  Bit Shift1 : hdlsllib/Logic and Bit Operations/Bit Shift  mode=Shift Left Logical  N=7
      settings: SourceProductName=HDL Coder  SourceProductBaseCode=HD
  Cast1 : DataTypeConversion  OutDataTypeStr=double
  Constant1 : Constant  Value=2
  Constant2 : Constant  Value=2
  Display{1..5} (5 alike) : Display
  Divide : Product  Inputs=*/
  Fix1 : Rounding  Operator=fix
  Gain : Gain  Gain=-1
  Gain1 : Gain  Gain=-1
  Minus : Sum  Inputs=-+
  Minus1 : Sum  Inputs=+-
  Minus2 : Sum
  Multiply : Product
  Multiply1 : Product
  Power : Math  Priority=5  Operator=pow  SaturateOnIntegerOverflow=on
  Power1 : Math  Priority=5  Operator=pow  SaturateOnIntegerOverflow=on
  Switch : Switch  Criteria=u2 > Threshold
  decoded : Outport
  wires:
  Bit Shift1/1 -> Minus/1
  [prec_pow] -> Multiply1/2
  [prec_pow] -> Divide/2
  Power1/1 -> [prec_pow]
  Constant2/1 -> Power1/1
  precision/1 -> [precision], Power1/2
  Cast1/1 -> Minus/2
  Divide/1 -> Fix1/1
  Switch/1 -> decoded/1, Display3/1
  Gain1/1 -> Switch/1
  Minus2/1 -> Switch/3, Gain1/1
  Multiply/1 -> Minus2/1
  [precision] -> Gain/1
  Power/1 -> Multiply/2
  Gain/1 -> Power/2
  Constant1/1 -> Power/1
  Minus1/1 -> Multiply/1, Display5/1
  Multiply1/1 -> Minus1/2
  Fix1/1 -> Multiply1/1, Display4/1, Minus2/2
  Minus/1 -> Minus1/1, Display2/1, Divide/1
  value/1 -> Bit Shift/1, Cast1/1
  Bit Shift/1 -> Display1/1, Switch/2, Bit Shift1/1

== system HANcoder_E407_CAN_COMM_TEST/HANcoder STM32 Target - E407-STM32 algorithm/Rx CAN/uint8_2float15 ==
  precision : Inport
  value : Inport  Port=2
  Bit Shift : hdlsllib/Logic and Bit Operations/Bit Shift  mode=Shift Right Logical  N=7
      settings: SourceProductName=HDL Coder  SourceProductBaseCode=HD
  Bit Shift1 : hdlsllib/Logic and Bit Operations/Bit Shift  mode=Shift Left Logical  N=7
      settings: SourceProductName=HDL Coder  SourceProductBaseCode=HD
  Cast1 : DataTypeConversion  OutDataTypeStr=double
  Constant1 : Constant  Value=2
  Constant2 : Constant  Value=2
  Display{1..5} (5 alike) : Display
  Divide : Product  Inputs=*/
  Fix1 : Rounding  Operator=fix
  Gain : Gain  Gain=-1
  Gain1 : Gain  Gain=-1
  Minus : Sum  Inputs=-+
  Minus1 : Sum  Inputs=+-
  Minus2 : Sum
  Multiply : Product
  Multiply1 : Product
  Power : Math  Priority=5  Operator=pow  SaturateOnIntegerOverflow=on
  Power1 : Math  Priority=5  Operator=pow  SaturateOnIntegerOverflow=on
  Switch : Switch  Criteria=u2 > Threshold
  decoded : Outport
  wires:
  Bit Shift1/1 -> Minus/1
  [prec_pow] -> Multiply1/2
  [prec_pow] -> Divide/2
  Power1/1 -> [prec_pow]
  Constant2/1 -> Power1/1
  precision/1 -> [precision], Power1/2
  Cast1/1 -> Minus/2
  Divide/1 -> Fix1/1
  Switch/1 -> decoded/1, Display3/1
  Gain1/1 -> Switch/1
  Minus2/1 -> Switch/3, Gain1/1
  Multiply/1 -> Minus2/1
  [precision] -> Gain/1
  Power/1 -> Multiply/2
  Gain/1 -> Power/2
  Constant1/1 -> Power/1
  Minus1/1 -> Multiply/1, Display5/1
  Multiply1/1 -> Minus1/2
  Fix1/1 -> Multiply1/1, Display4/1, Minus2/2
  Minus/1 -> Minus1/1, Display2/1, Divide/1
  value/1 -> Cast1/1, Bit Shift/1
  Bit Shift/1 -> Display1/1, Switch/2, Bit Shift1/1

== system HANcoder_E407_CAN_COMM_TEST/HANcoder STM32 Target - E407-STM32 algorithm/Rx CAN/uint8_2float16 ==
  precision : Inport
  value : Inport  Port=2
  Bit Shift : hdlsllib/Logic and Bit Operations/Bit Shift  mode=Shift Right Logical  N=7
      settings: SourceProductName=HDL Coder  SourceProductBaseCode=HD
  Bit Shift1 : hdlsllib/Logic and Bit Operations/Bit Shift  mode=Shift Left Logical  N=7
      settings: SourceProductName=HDL Coder  SourceProductBaseCode=HD
  Cast1 : DataTypeConversion  OutDataTypeStr=double
  Constant1 : Constant  Value=2
  Constant2 : Constant  Value=2
  Display{1..5} (5 alike) : Display
  Divide : Product  Inputs=*/
  Fix1 : Rounding  Operator=fix
  Gain : Gain  Gain=-1
  Gain1 : Gain  Gain=-1
  Minus : Sum  Inputs=-+
  Minus1 : Sum  Inputs=+-
  Minus2 : Sum
  Multiply : Product
  Multiply1 : Product
  Power : Math  Priority=5  Operator=pow  SaturateOnIntegerOverflow=on
  Power1 : Math  Priority=5  Operator=pow  SaturateOnIntegerOverflow=on
  Switch : Switch  Criteria=u2 > Threshold
  decoded : Outport
  wires:
  Bit Shift1/1 -> Minus/1
  [prec_pow] -> Multiply1/2
  [prec_pow] -> Divide/2
  Power1/1 -> [prec_pow]
  Constant2/1 -> Power1/1
  precision/1 -> [precision], Power1/2
  Cast1/1 -> Minus/2
  Divide/1 -> Fix1/1
  Switch/1 -> decoded/1, Display3/1
  Gain1/1 -> Switch/1
  Minus2/1 -> Switch/3, Gain1/1
  Multiply/1 -> Minus2/1
  [precision] -> Gain/1
  Power/1 -> Multiply/2
  Gain/1 -> Power/2
  Constant1/1 -> Power/1
  Minus1/1 -> Multiply/1, Display5/1
  Multiply1/1 -> Minus1/2
  Fix1/1 -> Multiply1/1, Display4/1, Minus2/2
  Minus/1 -> Minus1/1, Display2/1, Divide/1
  value/1 -> Bit Shift/1, Cast1/1
  Bit Shift/1 -> Display1/1, Switch/2, Bit Shift1/1

== system HANcoder_E407_CAN_COMM_TEST/HANcoder STM32 Target - E407-STM32 algorithm/Rx CAN/uint8_2float2 ==
  precision : Inport
  value : Inport  Port=2
  Bit Shift : hdlsllib/Logic and Bit Operations/Bit Shift  mode=Shift Right Logical  N=7
      settings: SourceProductName=HDL Coder  SourceProductBaseCode=HD
  Bit Shift1 : hdlsllib/Logic and Bit Operations/Bit Shift  mode=Shift Left Logical  N=7
      settings: SourceProductName=HDL Coder  SourceProductBaseCode=HD
  Cast1 : DataTypeConversion  OutDataTypeStr=double
  Constant1 : Constant  Value=2
  Constant2 : Constant  Value=2
  Display{1..5} (5 alike) : Display
  Divide : Product  Inputs=*/
  Fix1 : Rounding  Operator=fix
  Gain : Gain  Gain=-1
  Gain1 : Gain  Gain=-1
  Minus : Sum  Inputs=-+
  Minus1 : Sum  Inputs=+-
  Minus2 : Sum
  Multiply : Product
  Multiply1 : Product
  Power : Math  Priority=5  Operator=pow  SaturateOnIntegerOverflow=on
  Power1 : Math  Priority=5  Operator=pow  SaturateOnIntegerOverflow=on
  Switch : Switch  Criteria=u2 > Threshold
  decoded : Outport
  wires:
  Bit Shift1/1 -> Minus/1
  [prec_pow] -> Multiply1/2
  [prec_pow] -> Divide/2
  Power1/1 -> [prec_pow]
  Constant2/1 -> Power1/1
  precision/1 -> [precision], Power1/2
  Cast1/1 -> Minus/2
  Divide/1 -> Fix1/1
  Switch/1 -> decoded/1, Display3/1
  Gain1/1 -> Switch/1
  Minus2/1 -> Switch/3, Gain1/1
  Multiply/1 -> Minus2/1
  [precision] -> Gain/1
  Power/1 -> Multiply/2
  Gain/1 -> Power/2
  Constant1/1 -> Power/1
  Minus1/1 -> Multiply/1, Display5/1
  Multiply1/1 -> Minus1/2
  Fix1/1 -> Multiply1/1, Display4/1, Minus2/2
  Minus/1 -> Minus1/1, Display2/1, Divide/1
  value/1 -> Bit Shift/1, Cast1/1
  Bit Shift/1 -> Display1/1, Switch/2, Bit Shift1/1

== system HANcoder_E407_CAN_COMM_TEST/HANcoder STM32 Target - E407-STM32 algorithm/Rx CAN/uint8_2float3 ==
  precision : Inport
  value : Inport  Port=2
  Bit Shift : hdlsllib/Logic and Bit Operations/Bit Shift  mode=Shift Right Logical  N=7
      settings: SourceProductName=HDL Coder  SourceProductBaseCode=HD
  Bit Shift1 : hdlsllib/Logic and Bit Operations/Bit Shift  mode=Shift Left Logical  N=7
      settings: SourceProductName=HDL Coder  SourceProductBaseCode=HD
  Cast1 : DataTypeConversion  OutDataTypeStr=double
  Constant1 : Constant  Value=2
  Constant2 : Constant  Value=2
  Display{1..5} (5 alike) : Display
  Divide : Product  Inputs=*/
  Fix1 : Rounding  Operator=fix
  Gain : Gain  Gain=-1
  Gain1 : Gain  Gain=-1
  Minus : Sum  Inputs=-+
  Minus1 : Sum  Inputs=+-
  Minus2 : Sum
  Multiply : Product
  Multiply1 : Product
  Power : Math  Priority=5  Operator=pow  SaturateOnIntegerOverflow=on
  Power1 : Math  Priority=5  Operator=pow  SaturateOnIntegerOverflow=on
  Switch : Switch  Criteria=u2 > Threshold
  decoded : Outport
  wires:
  Bit Shift/1 -> Bit Shift1/1, Switch/2, Display1/1
  value/1 -> Cast1/1, Bit Shift/1
  Minus/1 -> Divide/1, Display2/1, Minus1/1
  Fix1/1 -> Minus2/2, Display4/1, Multiply1/1
  Multiply1/1 -> Minus1/2
  Minus1/1 -> Display5/1, Multiply/1
  Constant1/1 -> Power/1
  Gain/1 -> Power/2
  Power/1 -> Multiply/2
  [precision] -> Gain/1
  Multiply/1 -> Minus2/1
  Minus2/1 -> Gain1/1, Switch/3
  Gain1/1 -> Switch/1
  Switch/1 -> Display3/1, decoded/1
  Divide/1 -> Fix1/1
  Cast1/1 -> Minus/2
  precision/1 -> Power1/2, [precision]
  Constant2/1 -> Power1/1
  Power1/1 -> [prec_pow]
  [prec_pow] -> Divide/2
  [prec_pow] -> Multiply1/2
  Bit Shift1/1 -> Minus/1
